simulink model "TestingUSRPSimulink"  (R2019b)
settings: Solver=VariableStepAuto  StartTime=0.0  StopTime=6  RelTol=1e-3
undefined symbols (not defined in the file): serial
libraries: commsdrhw_v2 x2, instrumentlib x2
settings Model: SimulationMode=accelerator  EnablePacing=on  Creator=xngha  LastModifiedBy=Xongile

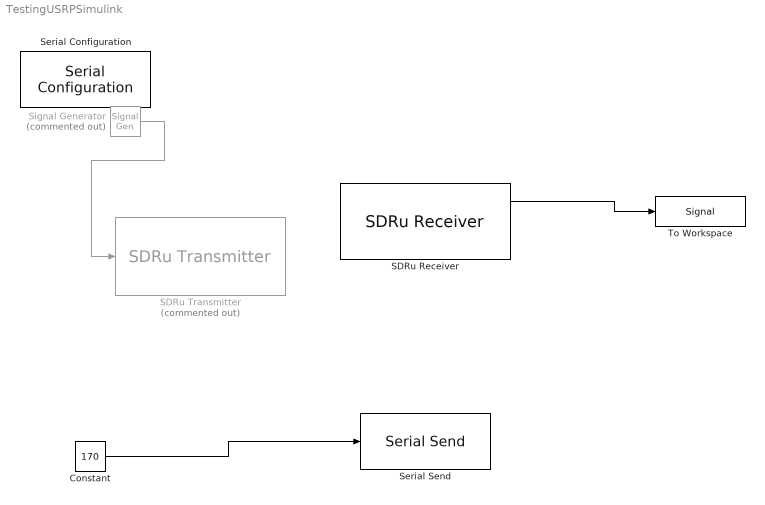
== system TestingUSRPSimulink ==
  Constant : Constant  Value=170  OutDataTypeStr=uint8  SampleTime=1
  SDRu Receiver : commsdrhw_v2/SDRu Receiver  rxtx=rx  initializeIPAddress=0  devMap=10  USRP2_IP=192.168.10.5  USRP_IP_X300=192.168.10.2  USRP_IP_X310=192.168.10.2  USRP_serialNumB210=3136D21  platform=N200/N210/USRP2  prevPlatform=N200/N210/USRP2  lastIPAddressPopup=192.168.10.2  USRP_ID=192.168.10.5  LastIPAddress=192.168.10.2  ChannelMapping=1  centerFrequencySrc=Dialog  centerFrequency=0  loOffsetSrc=Dialog  loOffset=0  gainSrc=Dialog  gain=4  PPSSource=Internal  clockSource=Internal  masterClkRateParam=100e6  masterClkRateB200=32e6  masterClkRateB210=32e6  masterClkRateX300=200e6  masterClkRateX310=200e6  masterClkRate=100e6  decimInterpSrc=Dialog  decimInterpPort=512  lastDecimSource=Dialog  decimInterp=10  USRP2_IP_NUM=[49 57 50 46 49 54 56 46 49 48 46 53]  sampleRate=10000000  sampleTime=1e-07  TransportDataType=int8  overrunUnderrunPort=off  outputDatatype=single  frameLength=1000  HOST_DATA_PORT=0  HOST_CONTROL_PORT=0  USRP2_DATA_PORT=0  USRP2_CONTROL_PORT=0  bufferMode=Continuous streaming  EnableBurstMode=off  NumFramesInBurst=10
      settings: SourceProductName=Communications Toolbox Support Package for USRP Radio  SourceProductBaseCode=USRP
  SDRu Transmitter : commsdrhw_v2/SDRu Transmitter  Commented=on  rxtx=tx  initializeIPAddress=0  devMap=0  USRP2_IP=192.168.10.5  USRP_IP_X300=192.168.10.2  USRP_IP_X310=192.168.10.2  USRP_serialNumB200=No devices found  USRP_serialNumB210=No devices found  platform=N200/N210/USRP2  prevPlatform=N200/N210/USRP2  lastIPAddressPopup=192.168.10.2  USRP_ID=192.168.10.5  LastIPAddress=192.168.10.2  ChannelMapping=1  centerFrequencySrc=Dialog  centerFrequency=0  loOffsetSrc=Dialog  loOffset=0  gainSrc=Dialog  gain=8  PPSSource=Internal  clockSource=Internal  masterClkRateParam=100e6  masterClkRateB200=32e6  masterClkRateB210=32e6  masterClkRateX300=120e6  masterClkRateX310=120e6  decimInterpSrc=Dialog  lastDecimSource=Dialog  decimInterp=512  USRP2_IP_NUM=[49 57 50 46 49 54 56 46 49 48 46 53]  frameLength=362  sampleRate=195312.5  TransportDataType=int16  outputDatatype=Same as transport data type  overrunUnderrunPort=off  sampleTime=5.12e-06  dboardInfo=|  HOST_DATA_PORT=30000  HOST_CONTROL_PORT=30001  USRP2_DATA_PORT=32769  USRP2_CONTROL_PORT=32768  bufferMode=Continuous streaming  EnableBurstMode=off  NumFramesInBurst=100
      | dbid: 0
      |           dbName: 'no db found'
      |          freqMin: 0
      |          freqMax: 0
      |          gainMin: 0
      |          gainMax: 0
      |     gainStepSize: 0
      settings: SourceProductName=Communications Toolbox Support Package for USRP Radio  SourceProductBaseCode=USRP
  Serial Configuration : instrumentlib/Serial Configuration  Priority=-200000  ComPortMenu=COM3  ComPort=COM3  ObjConstructor=serial('COM3');  BaudRate=9600  DataBits=8  Parity=none  StopBits=1  FlowControl=none  Timeout=10  ByteOrder=LittleEndian
  Serial Send : instrumentlib/Serial Send  ComPortMenu=COM3  ComPort=COM3  ObjConstructor=serial('COM3');  Terminator=<none>  EnableBlockingMode=on
  Signal Generator : SignalGenerator  Commented=on  Amplitude=0.7  Frequency=1e3  VectorParams1D=off
  To Workspace : ToWorkspace  VariableName=Signal  SaveFormat=Timeseries  SampleTime=-1
  wires:
  SDRu Receiver/1 -> To Workspace/1
  Signal Generator/1 -> SDRu Transmitter/1
  Constant/1 -> Serial Send/1
